simulink model "imu_acceleration"  (R2023b)
settings: Solver=VariableStepAuto  StartTime=0.0  StopTime=2  RelTol=1e-3
libraries: simulink x1, sensors_subsystems x1
settings Model: Creator=brent  LastModifiedBy=brent

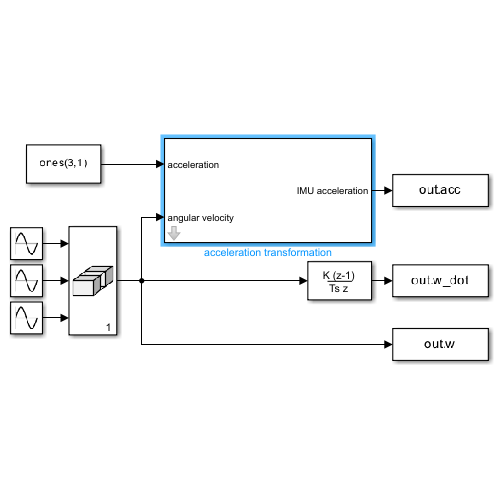
[thumbnail: Simulink's stored preview of the top-level diagram]
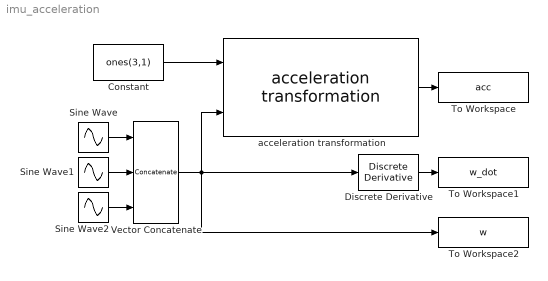
== system imu_acceleration ==
  Constant : Constant  Value=ones(3,1)
  Discrete Derivative : simulink/Discrete/Discrete Derivative  gainval=1.0  ICPrevScaledInput=0.0  OutMin=[]  OutMax=[]  OutDataType=fixdt(1, 16)  OutScaling=2^-10  DoSatur=off
  Sine Wave : Sin  SampleTime=0
  Sine Wave1 : Sin  SampleTime=0
  Sine Wave2 : Sin  SampleTime=0
  To Workspace : ToWorkspace  VariableName=acc  SampleTime=-1
  To Workspace1 : ToWorkspace  VariableName=w_dot  SampleTime=-1
  To Workspace2 : ToWorkspace  VariableName=w  SampleTime=-1
  Vector Concatenate : Concatenate  NumInputs=3  Mode=Multidimensional array
  acceleration transformation : sensors_subsystems/acceleration transformation  pos=IMU.position.value  angles=IMU.orientation.value
      settings: SourceProductName=Sensors library
  wires:
  Constant/1 -> acceleration transformation/1
  acceleration transformation/1 -> To Workspace/1
  Discrete Derivative/1 -> To Workspace1/1
  Sine Wave/1 -> Vector Concatenate/1
  Sine Wave1/1 -> Vector Concatenate/2
  Sine Wave2/1 -> Vector Concatenate/3
  Vector Concatenate/1 -> To Workspace2/1, Discrete Derivative/1, acceleration transformation/2
